simulink model "QUESTION2"  (R2020a)
settings: Solver=VariableStepAuto  StartTime=0.0  StopTime=10.0  RelTol=1e-3
model workspace (MAT data in the model file):
  b1 = Simulink.Parameter
  b1.Value = 350
  b1.DataType = 'auto'
  b1.Dimensions = [1 1]
  k1 = Simulink.Parameter
  k1.Value = 50000
  k1.DataType = 'auto'
  k1.Dimensions = [1 1]
  k2 = Simulink.Parameter
  k2.Value = 50000
  k2.DataType = 'auto'
  k2.Dimensions = [1 1]
  m1 = Simulink.Parameter
  m1.Value = 2500
  m1.DataType = 'auto'
  m1.Dimensions = [1 1]
  m2 = Simulink.Parameter
  m2.Value = 320
  m2.DataType = 'auto'
  m2.Dimensions = [1 1]
undefined symbols (not defined in the file): b
settings Model: OrderedModelArguments=off  Creator=anjal  LastModifiedBy=anjal

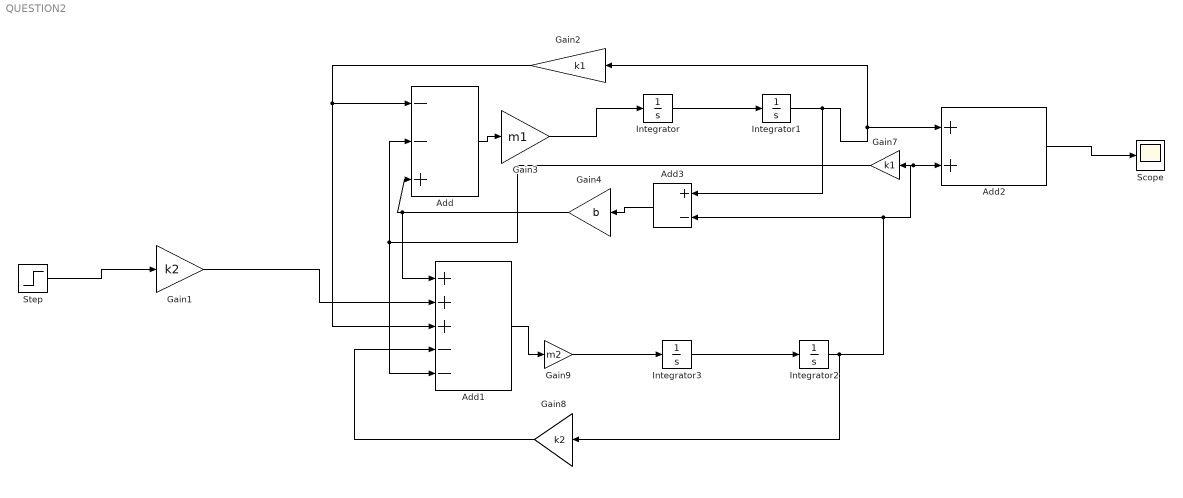
== system QUESTION2 ==
  Add : Sum  Inputs=--+
  Add1 : Sum  Inputs=+++--
  Add2 : Sum
  Add3 : Sum  Inputs=+-
  Gain1 : Gain  Gain=k2
  Gain2 : Gain  Gain=k1
  Gain3 : Gain  Gain=m1
  Gain4 : Gain  Gain=b
  Gain7 : Gain  Gain=k1
  Gain8 : Gain  Gain=k2
  Gain9 : Gain  Gain=m2
  Integrator{,1..3} (4 alike) : Integrator
  Scope : Scope
  Step : Step  Before=0.01  After=5  SampleTime=0
  wires:
  Gain7/1 -> Add/2, Add1/5
  Gain3/1 -> Integrator/1
  Integrator2/1 -> Gain8/1, Add3/2, Gain7/1, Add2/2
  Gain8/1 -> Add1/4
  Gain9/1 -> Integrator3/1
  Gain4/1 -> Add1/1, Add/3
  Gain2/1 -> Add/1, Add1/3
  Add1/1 -> Gain9/1
  Add2/1 -> Scope/1
  Step/1 -> Gain1/1
  Gain1/1 -> Add1/2
  Integrator/1 -> Integrator1/1
  Add/1 -> Gain3/1
  Integrator3/1 -> Integrator2/1
  Add3/1 -> Gain4/1
  Integrator1/1 -> Add3/1, Gain2/1, Add2/1
